simulink model "arduio_motor_control"  (R2015b)
settings: Solver=FixedStepDiscrete  SolverMode=SingleTasking  StartTime=0.0  StopTime=inf  RelTol=1e-3
libraries: arduinolib x9
settings Model: SimulationMode=external  ExtModeTrigDuration=2  Creator=Jordan  LastModifiedBy=Jordan
settings OptimizationCC: OptimizeModelRefInitCode=on  LifeSpan=1  MaxStackSize=64
settings HardwareCC: ProdBitPerPointer=32  ProdLargestAtomicInteger=Long  ProdLargestAtomicFloat=Double  ProdWordSize=32  ProdHWDeviceType=ARM Compatible->ARM Cortex
settings RTWCC: SystemTargetFile=ert.tlc  TemplateMakefile=ert_default_tmf  Description=Embedded Coder  Toolchain=Arduino ARM v1.6.1  BuildConfiguration=Faster Runs
settings CodeAppCC: IgnoreCustomStorageClasses=off

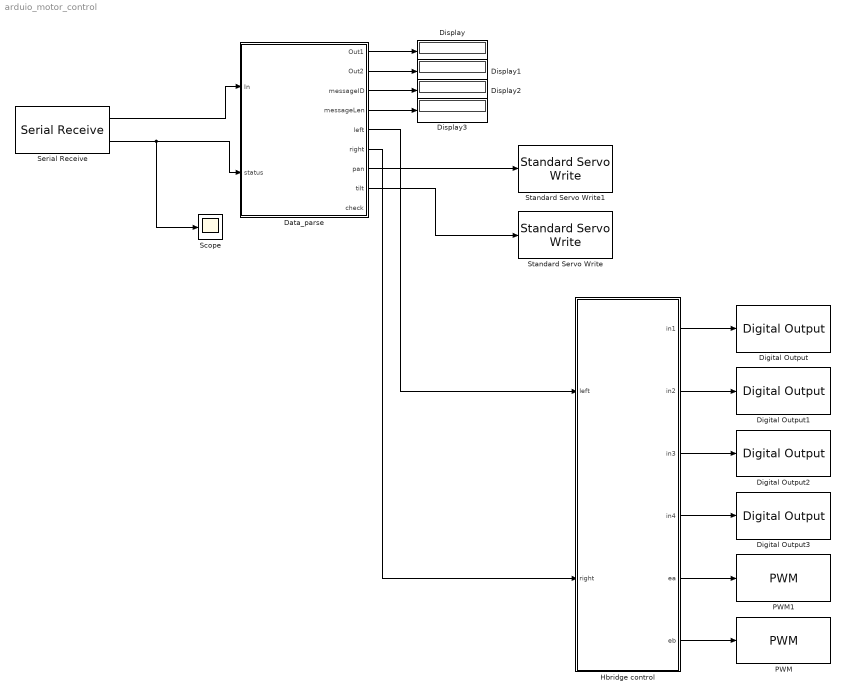
== system arduio_motor_control ==
  Data_parse : Subsystem
  Digital Output : arduinolib/Digital Output  pinNumber=8  blockPlatform=arduino
  Digital Output1 : arduinolib/Digital Output  pinNumber=7  blockPlatform=arduino
  Digital Output2 : arduinolib/Digital Output  pinNumber=13  blockPlatform=arduino
  Digital Output3 : arduinolib/Digital Output  pinNumber=12  blockPlatform=arduino
  Display{,1..3} (4 alike) : Display
  Hbridge control : MATLAB Function  TreatAsAtomicUnit=on
  PWM : arduinolib/PWM  pinNumber=11  blockPlatform=arduino
  PWM1 : arduinolib/PWM  pinNumber=6  blockPlatform=arduino
  Scope : Scope
  Serial Receive : arduinolib/Serial Receive  portNumber=1  showOutStatus=on  sampleTime=.001  blockPlatform=arduino
  Standard Servo Write : arduinolib/Standard Servo Write  pinNumber=5  blockPlatform=arduino
  Standard Servo Write1 : arduinolib/Standard Servo Write  pinNumber=3  blockPlatform=arduino
  wires:
  Serial Receive/1 -> Data_parse/1(In)
  Serial Receive/2 -> Scope/1, Data_parse/2(status)
  Data_parse/1(Out1) -> Display/1
  Data_parse/2(Out2) -> Display1/1
  Data_parse/3(messageID) -> Display2/1
  Data_parse/4(messageLen) -> Display3/1
  Data_parse/5(left) -> Hbridge control/1(left)
  Data_parse/6(right) -> Hbridge control/2(right)
  Data_parse/7(pan) -> Standard Servo Write1/1
  Data_parse/8(tilt) -> Standard Servo Write/1
  Hbridge control/1(in1) -> Digital Output/1
  Hbridge control/2(in2) -> Digital Output1/1
  Hbridge control/3(in3) -> Digital Output2/1
  Hbridge control/4(in4) -> Digital Output3/1
  Hbridge control/5(ea) -> PWM1/1
  Hbridge control/6(eb) -> PWM/1

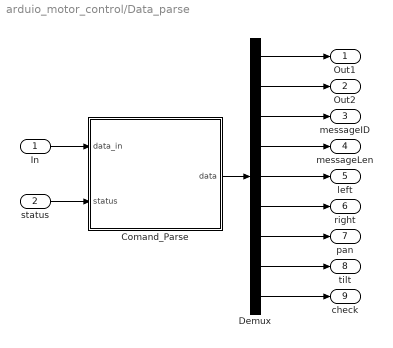
== system arduio_motor_control/Data_parse ==
  In : Inport
  status : Inport  Port=2
  Comand_Parse : Stateflow chart  TreatAsAtomicUnit=on
  Demux : Demux  Outputs=9
  Out1 : Outport
  Out2 : Outport  Port=2
  messageID : Outport  Port=3
  messageLen : Outport  Port=4
  left : Outport  Port=5
  right : Outport  Port=6
  pan : Outport  Port=7
  tilt : Outport  Port=8
  check : Outport  Port=9
  wires:
  In/1 -> Comand_Parse/1(data_in)
  status/1 -> Comand_Parse/2(status)
  Comand_Parse/1(data) -> Demux/1
  Demux/1 -> Out1/1
  Demux/2 -> Out2/1
  Demux/3 -> messageID/1
  Demux/4 -> messageLen/1
  Demux/5 -> left/1
  Demux/6 -> right/1
  Demux/7 -> pan/1
  Demux/8 -> tilt/1
  Demux/9 -> check/1

== matlab function arduio_motor_control/Hbridge control ==
  data: left input; in1 output; right input; in2 output; in3 output; in4 output; ea output; eb output
function [in1, in2, in3, in4, ea, eb]  = fcn(left,right)
%#codegen
if left <= 127;
    in1 = true;
    in2 = false;
    ea = uint8(left * 2);
else 
    in1 = false;
    in2 = true;
    ea = uint8((left -127) *2);
end

 if right <= 127;
    in3 = true;
    in4 = false;
    eb = uint8(left * 2);
else 
    in3 = false;
    in4 = true;
    eb = uint8((left -127) *2);
end

== stateflow chart arduio_motor_control/Data_parse/Comand_Parse ==
  settings: updateMethod=DISCRETE  sampleTime=.001
  state idel
    entry:
    cnt = uint8(0);
    during:
  state Get_byte
    entry: data(cnt) = data_in;
  state wait
  (default) -> idel : {data = uint8([0;0;0;0;0;0;0;0;0]);}
  wait -> idel [order 1] : [cnt == uint8(9)]
  idel -> Get_byte : [status == true]
      | {cnt = cnt +1;}
  wait -> Get_byte [order 2] : [status == true]
      | {cnt = cnt +1;}
  Get_byte -> wait
  data: data_in input; status input; data output; cnt local
